simulink library "ComponentLibrary"  (R2017b)
settings: Solver=VariableStepAuto  StartTime=0.0  StopTime=10.0  RelTol=1e-3
undefined symbols (not defined in the file): pelvisPosition, pelvisVelocity, X, Y, Z
libraries: xpcethercatlib x79, sm_lib x21, nesl_utility x13, slrtlib x3, ComponentLibrary x2
(part 2 of 2)

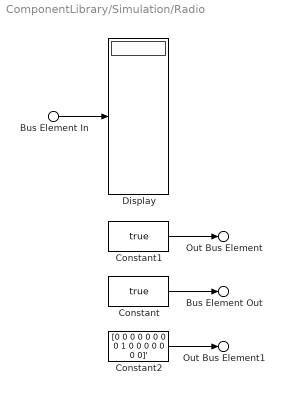
== system ComponentLibrary/Simulation/Radio ==
  Bus Element In : Inport  PortName=InBus  Element=channel
  Constant : Constant  Value=true  OutDataTypeStr=boolean
  Constant1 : Constant  Value=true  OutDataTypeStr=boolean
  Constant2 : Constant  Value=[0 0 0 0 0 0 0 0 1 0 0 0 0 0 0 0]'
  Display : Display
  Out Bus Element : Outport  PortName=OutBus  Element=radioReceiverSignalGood
  Bus Element Out : Outport  PortName=OutBus  Element=receiverMedullaSignalGood
  Out Bus Element1 : Outport  PortName=OutBus  Element=channel
  wires:
  Constant1/1 -> Out Bus Element/1
  Constant2/1 -> Out Bus Element1/1
  Constant/1 -> Bus Element Out/1
  Bus Element In/1 -> Display/1

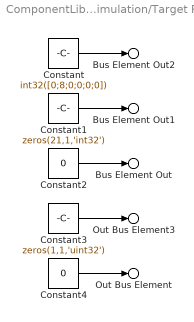
== system ComponentLibrary/Simulation/Target PC ==
  Constant : Constant  Value=int32([0;8;0;0;0;0])
  Constant1 : Constant  Value=zeros(21,1,'int32')
  Constant2 : Constant  Value=0
  Constant3 : Constant  Value=zeros(1,1,'uint32')
  Constant4 : Constant  Value=0
  Bus Element Out2 : Outport  PortName=OutBus  Element=etherCatStatus
  Bus Element Out1 : Outport  PortName=OutBus  Element=etherCatNotifications
  Bus Element Out : Outport  PortName=OutBus  Element=taskExecutionTime
  Out Bus Element3 : Outport  PortName=OutBus  Element=overloadCounter
  Out Bus Element : Outport  PortName=OutBus  Element=cpuTemperature
  wires:
  Constant/1 -> Bus Element Out2/1
  Constant1/1 -> Bus Element Out1/1
  Constant2/1 -> Bus Element Out/1
  Constant4/1 -> Out Bus Element/1
  Constant3/1 -> Out Bus Element3/1

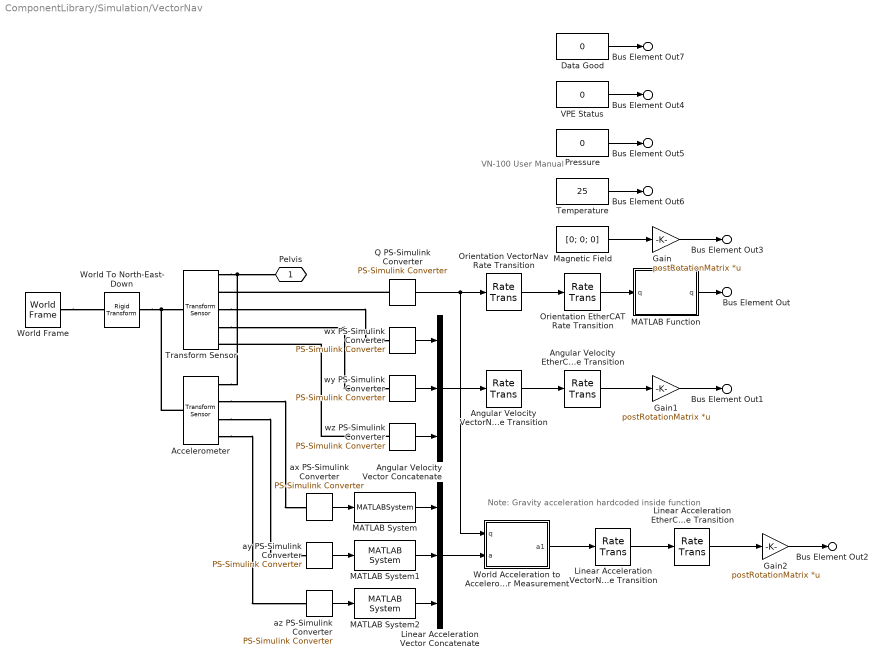
== system ComponentLibrary/Simulation/VectorNav ==
  note: Note: Gravity acceleration hardcoded inside function
  note: VN-100 User Manual
  Accelerometer : sm_lib/Frames and Transforms/Transform Sensor  MeasurementFrame=Base  SenseAngle=off  SenseAxis=off  SenseAngle1=off  SenseAngle2=off  SenseAngle3=off  SenseQ=off  SenseR=off  SenseOmegaX=off  SenseOmegaY=off  SenseOmegaZ=off  SenseOmega1=off  SenseOmega2=off  SenseOmega3=off  SenseQDot=off  SenseRDot=off  SenseAlphaX=off  SenseAlphaY=off  SenseAlphaZ=off  SenseAlpha1=off  SenseAlpha2=off  SenseAlpha3=off  SenseQDDot=off  SenseRDDot=off  SenseX=off  SenseY=off  SenseZ=off  SenseRad=off  SenseAzim=off  SenseDist=off  SenseInc=off  SenseXDot=off  SenseYDot=off  SenseZDot=off  SenseRadDot=off  SenseAzimDot=off  SenseDistDot=off  SenseIncDot=off  SenseXDDot=on  SenseYDDot=on  SenseZDDot=on  SenseRadDDot=off  SenseAzimDDot=off  SenseDistDDot=off  SenseIncDDot=off
  Angular Velocity EtherCAT Rate Transition : RateTransition  Deterministic=off  OutPortSampleTimeOpt=Inherit
  Angular Velocity Vector Concatenate : Concatenate  NumInputs=3
  Angular Velocity VectorNav Rate Transition : RateTransition  Deterministic=off  OutPortSampleTime=VectorNavModule.sampleTime
  Data Good : Constant  Value=0  OutDataTypeStr=boolean
  Gain : Gain  Gain=postRotationMatrix  Multiplication=Matrix(K*u)
  Gain1 : Gain  Gain=postRotationMatrix  Multiplication=Matrix(K*u)
  Gain2 : Gain  Gain=postRotationMatrix  Multiplication=Matrix(K*u)
  Linear Acceleration EtherCAT Rate Transition : RateTransition  Deterministic=off  InitialCondition=[0; 0; 0]  OutPortSampleTimeOpt=Inherit
  Linear Acceleration Vector Concatenate : Concatenate  NumInputs=3
  Linear Acceleration VectorNav Rate Transition : RateTransition  Deterministic=off  InitialCondition=[0; 0; 0]  OutPortSampleTime=VectorNavModule.sampleTime
  MATLAB Function : MATLAB Function  TreatAsAtomicUnit=on
  MATLAB System : MATLABSystem  System=FilterSystem  a=[1 -0.8]  b=0.2  SimulateUsing=Code generation
      mask Type: FilterSystem
      mask Display: disp('Filter');
  MATLAB System1 : ComponentLibrary/Simulation/VectorNav/MATLAB System  a=[1 -0.8]  b=0.2  SimulateUsing=Code generation
  MATLAB System2 : ComponentLibrary/Simulation/VectorNav/MATLAB System  a=[1 -0.8]  b=0.2  SimulateUsing=Code generation
  Magnetic Field : Constant  Value=[0; 0; 0]
  Orientation EtherCAT Rate Transition : RateTransition  Deterministic=off  InitialCondition=[0; 0; 0; 1]  OutPortSampleTimeOpt=Inherit
  Orientation VectorNav Rate Transition : RateTransition  Deterministic=off  InitialCondition=[0; 0; 0; 1]  OutPortSampleTime=VectorNavModule.sampleTime
  Pressure : Constant  Value=0
  Q PS-Simulink Converter : nesl_utility/PS-Simulink Converter  PhysicalDomain=network_engine_domain  SubClassName=ps_output  LeftPortType=input  RightPortType=output  PseudoPeriodic=off  Frequencies=[]  Unit=1  AffineConversion=off
  Temperature : Constant  Value=25
  Transform Sensor : sm_lib/Frames and Transforms/Transform Sensor  MeasurementFrame=Follower  SenseAngle=off  SenseAxis=off  SenseAngle1=off  SenseAngle2=off  SenseAngle3=off  SenseQ=on  SenseR=off  SenseOmegaX=on  SenseOmegaY=on  SenseOmegaZ=on  SenseOmega1=off  SenseOmega2=off  SenseOmega3=off  SenseQDot=off  SenseRDot=off  SenseAlphaX=off  SenseAlphaY=off  SenseAlphaZ=off  SenseAlpha1=off  SenseAlpha2=off  SenseAlpha3=off  SenseQDDot=off  SenseRDDot=off  SenseX=off  SenseY=off  SenseZ=off  SenseRad=off  SenseAzim=off  SenseDist=off  SenseInc=off  SenseXDot=off  SenseYDot=off  SenseZDot=off  SenseRadDot=off  SenseAzimDot=off  SenseDistDot=off  SenseIncDot=off  SenseXDDot=off  SenseYDDot=off  SenseZDDot=off  SenseRadDDot=off  SenseAzimDDot=off  SenseDistDDot=off  SenseIncDDot=off
  VPE Status : Constant  Value=0  OutDataTypeStr=uint16
  World Acceleration to Accelerometer Measurement : MATLAB Function  TreatAsAtomicUnit=on
  World Frame : sm_lib/Frames and Transforms/World Frame
  World To North-East-Down : sm_lib/Frames and Transforms/Rigid Transform  TranslationMethod=None  TranslationStandardOffset=0  TranslationLengthUnit=m  TranslationStandardAxis=+Z  TranslationCartesianOffset=[0 0 0]  TranslationROffset=0  TranslationROffsetUnits=m  TranslationZOffset=0  TranslationZOffsetUnits=m  TranslationThetaOffset=0  TranslationThetaOffsetUnits=deg  RotationMethod=StandardAxis  RotationAngleUnits=deg  RotationStandardAxis=+X  RotationAngle=180  RotationArbitraryAxis=[0 0 1]  FollAlignAxisA=+X  BaseAlignAxisA=+Y  FollAlignAxisB=+Y  BaseAlignAxisB=+Z  RotationSequenceAxes=FollowerAxes  RotationSequence=XYX  RotationSequenceAngles=[0 0 0]  RotationSequenceAnglesUnits=deg  RotationMatrix=[1 0 0; 0 1 0; 0 0 1]
  ax PS-Simulink Converter : nesl_utility/PS-Simulink Converter  PhysicalDomain=network_engine_domain  SubClassName=ps_output  LeftPortType=input  RightPortType=output  PseudoPeriodic=off  Frequencies=[]  Unit=m/s/s  AffineConversion=off
  ay PS-Simulink Converter : nesl_utility/PS-Simulink Converter  PhysicalDomain=network_engine_domain  SubClassName=ps_output  LeftPortType=input  RightPortType=output  PseudoPeriodic=off  Frequencies=[]  Unit=m/s/s  AffineConversion=off
  az PS-Simulink Converter : nesl_utility/PS-Simulink Converter  PhysicalDomain=network_engine_domain  SubClassName=ps_output  LeftPortType=input  RightPortType=output  PseudoPeriodic=off  Frequencies=[]  Unit=m/s/s  AffineConversion=off
  wx PS-Simulink Converter : nesl_utility/PS-Simulink Converter  PhysicalDomain=network_engine_domain  SubClassName=ps_output  LeftPortType=input  RightPortType=output  PseudoPeriodic=off  Frequencies=[]  Unit=1  AffineConversion=off
  wy PS-Simulink Converter : nesl_utility/PS-Simulink Converter  PhysicalDomain=network_engine_domain  SubClassName=ps_output  LeftPortType=input  RightPortType=output  PseudoPeriodic=off  Frequencies=[]  Unit=1  AffineConversion=off
  wz PS-Simulink Converter : nesl_utility/PS-Simulink Converter  PhysicalDomain=network_engine_domain  SubClassName=ps_output  LeftPortType=input  RightPortType=output  PseudoPeriodic=off  Frequencies=[]  Unit=1  AffineConversion=off
  Pelvis : PMIOPort  Port=1  Side=Left
  Bus Element Out7 : Outport  PortName=OutBus  Element=dataGood
  Bus Element Out4 : Outport  PortName=OutBus  Element=vpeStatus
  Bus Element Out5 : Outport  PortName=OutBus  Element=pressure
  Bus Element Out6 : Outport  PortName=OutBus  Element=temperature
  Bus Element Out3 : Outport  PortName=OutBus  Element=magneticField
  Bus Element Out1 : Outport  PortName=OutBus  Element=angularVelocity
  Bus Element Out2 : Outport  PortName=OutBus  Element=linearAcceleration
  Bus Element Out : Outport  PortName=OutBus  Element=orientation
  wires:
  Angular Velocity VectorNav Rate Transition/1 -> Angular Velocity EtherCAT Rate Transition/1
  wz PS-Simulink Converter/1 -> Angular Velocity Vector Concatenate/3
  az PS-Simulink Converter/1 -> MATLAB System2/1
  wx PS-Simulink Converter/1 -> Angular Velocity Vector Concatenate/1
  ax PS-Simulink Converter/1 -> MATLAB System/1
  VPE Status/1 -> Bus Element Out4/1
  Orientation EtherCAT Rate Transition/1 -> MATLAB Function/1("q ")
  Q PS-Simulink Converter/1 -> World Acceleration to Accelerometer Measurement/1(q), Orientation VectorNav Rate Transition/1
  Temperature/1 -> Bus Element Out6/1
  wy PS-Simulink Converter/1 -> Angular Velocity Vector Concatenate/2
  Angular Velocity EtherCAT Rate Transition/1 -> Gain1/1
  Orientation VectorNav Rate Transition/1 -> Orientation EtherCAT Rate Transition/1
  Linear Acceleration EtherCAT Rate Transition/1 -> Gain2/1
  Linear Acceleration VectorNav Rate Transition/1 -> Linear Acceleration EtherCAT Rate Transition/1
  Data Good/1 -> Bus Element Out7/1
  ay PS-Simulink Converter/1 -> MATLAB System1/1
  Magnetic Field/1 -> Gain/1
  Angular Velocity Vector Concatenate/1 -> Angular Velocity VectorNav Rate Transition/1
  Pressure/1 -> Bus Element Out5/1
  Gain/1 -> Bus Element Out3/1
  Gain1/1 -> Bus Element Out1/1
  MATLAB Function/1(q) -> Bus Element Out/1
  MATLAB System/1 -> Linear Acceleration Vector Concatenate/1
  MATLAB System1/1 -> Linear Acceleration Vector Concatenate/2
  MATLAB System2/1 -> Linear Acceleration Vector Concatenate/3
  Gain2/1 -> Bus Element Out2/1
  World Acceleration to Accelerometer Measurement/1(a1) -> Linear Acceleration VectorNav Rate Transition/1
  Linear Acceleration Vector Concatenate/1 -> World Acceleration to Accelerometer Measurement/2(a)
  connections:
  Transform Sensor/RConn4 -- wy PS-Simulink Converter/LConn1
  World To North-East-Down/RConn1 -- Accelerometer/LConn1 -- Transform Sensor/LConn1
  Accelerometer/RConn3 -- ay PS-Simulink Converter/LConn1
  World Frame/RConn1 -- World To North-East-Down/LConn1
  Q PS-Simulink Converter/LConn1 -- Transform Sensor/RConn2
  Accelerometer/RConn2 -- ax PS-Simulink Converter/LConn1
  Transform Sensor/RConn1 -- Pelvis/RConn1 -- Accelerometer/RConn1
  Accelerometer/RConn4 -- az PS-Simulink Converter/LConn1
  Transform Sensor/RConn3 -- wx PS-Simulink Converter/LConn1
  wz PS-Simulink Converter/LConn1 -- Transform Sensor/RConn5

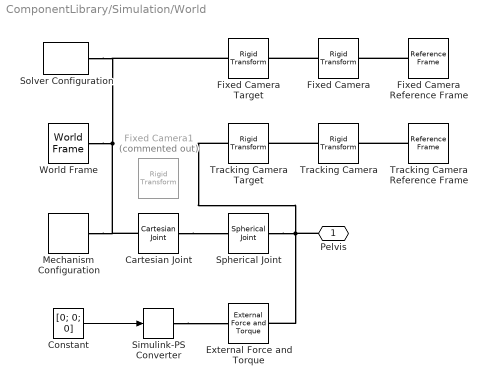
== system ComponentLibrary/Simulation/World ==
  Cartesian Joint : sm_lib/Joints/Cartesian Joint  SenseConstraintForce=off  SenseConstraintForceX=off  SenseConstraintForceY=off  SenseConstraintForceZ=off  SenseConstraintTorque=off  SenseConstraintTorqueX=off  SenseConstraintTorqueY=off  SenseConstraintTorqueZ=off  SenseTotalForce=off  SenseTotalForceX=off  SenseTotalForceY=off  SenseTotalForceZ=off  SenseTotalTorque=off  SenseTotalTorqueX=off  SenseTotalTorqueY=off  SenseTotalTorqueZ=off  CompositeWrenchDir=FollowerOnBase  CompositeWrenchFrame=BaseFrame  PxEquilibriumPosition=0  PxEquilibriumPositionUnits=m  PxSpringStiffness=0  PxSpringStiffnessUnits=N/m  PxDampingCoefficient=0  PxDampingCoefficientUnits=N/(m/s)  PxTorqueActuationMode=NoTorque  PxMotionActuationMode=ComputedMotion  PxSensePosition=off  PxSenseVelocity=off  PxSenseAcceleration=off  PxSenseTorqueForce=off  PxPositionTargetSpecify=on  PxPositionTargetPriority=High  PxPositionTargetValue=pelvisPosition(1)  PxPositionTargetValueUnits=m  PxVelocityTargetSpecify=on  PxVelocityTargetPriority=High  PxVelocityTargetValue=pelvisVelocity(1)  PxVelocityTargetValueUnits=m/s  PyEquilibriumPosition=0  PyEquilibriumPositionUnits=m  PySpringStiffness=0  PySpringStiffnessUnits=N/m  PyDampingCoefficient=0  PyDampingCoefficientUnits=N/(m/s)  PyTorqueActuationMode=NoTorque  PyMotionActuationMode=ComputedMotion  PySensePosition=off  PySenseVelocity=off  PySenseAcceleration=off  PySenseTorqueForce=off  PyPositionTargetSpecify=on  PyPositionTargetPriority=High  PyPositionTargetValue=pelvisPosition(2)  PyPositionTargetValueUnits=m  PyVelocityTargetSpecify=on  PyVelocityTargetPriority=High  PyVelocityTargetValue=pelvisVelocity(2)  PyVelocityTargetValueUnits=m/s  PzEquilibriumPosition=pelvisPosition(3)  PzEquilibriumPositionUnits=m  PzSpringStiffness=5000  PzSpringStiffnessUnits=N/m  PzDampingCoefficient=500  PzDampingCoefficientUnits=N/(m/s)  PzTorqueActuationMode=NoTorque  PzMotionActuationMode=ComputedMotion  PzSensePosition=off  PzSenseVelocity=off  PzSenseAcceleration=off  PzSenseTorqueForce=off  PzPositionTargetSpecify=on  PzPositionTargetPriority=High  PzPositionTargetValue=pelvisPosition(3)  PzPositionTargetValueUnits=m  PzVelocityTargetSpecify=on  PzVelocityTargetPriority=High  PzVelocityTargetValue=pelvisVelocity(3)  PzVelocityTargetValueUnits=m/s
  Constant : Constant  Value=[0; 0; 0]
  External Force and Torque : sm_lib/Forces and Torques/External Force and Torque  ForceResolutionFrame=World  EnableForceX=off  EnableForceY=off  EnableForceZ=off  EnableForce=on  TorqueResolutionFrame=AttachedFrame  EnableTorqueX=off  EnableTorqueY=off  EnableTorqueZ=off  EnableTorque=off
  Fixed Camera : sm_lib/Frames and Transforms/Rigid Transform  TranslationMethod=Cartesian  TranslationStandardOffset=0  TranslationLengthUnit=m  TranslationStandardAxis=+Z  TranslationCartesianOffset=[1.5 -1.5 0.5]  TranslationROffset=0  TranslationROffsetUnits=m  TranslationZOffset=0  TranslationZOffsetUnits=m  TranslationThetaOffset=0  TranslationThetaOffsetUnits=deg  RotationMethod=None  RotationAngleUnits=deg  RotationStandardAxis=+Z  RotationAngle=0.0  RotationArbitraryAxis=[0 0 1]  FollAlignAxisA=+X  BaseAlignAxisA=+Y  FollAlignAxisB=+Y  BaseAlignAxisB=+Z  RotationSequenceAxes=FollowerAxes  RotationSequence=XYX  RotationSequenceAngles=[0 0 0]  RotationSequenceAnglesUnits=deg  RotationMatrix=[1 0 0; 0 1 0; 0 0 1]
  Fixed Camera1 : sm_lib/Frames and Transforms/Rigid Transform  Commented=on  TranslationMethod=Cartesian  TranslationStandardOffset=0  TranslationLengthUnit=m  TranslationStandardAxis=+Z  TranslationCartesianOffset=[pelvisPosition(1),pelvisPosition(2),pelvisPosition(3)]  TranslationROffset=0  TranslationROffsetUnits=m  TranslationZOffset=0  TranslationZOffsetUnits=m  TranslationThetaOffset=0  TranslationThetaOffsetUnits=deg  RotationMethod=None  RotationAngleUnits=deg  RotationStandardAxis=+Z  RotationAngle=0.0  RotationArbitraryAxis=[0 0 1]  FollAlignAxisA=+X  BaseAlignAxisA=+Y  FollAlignAxisB=+Y  BaseAlignAxisB=+Z  RotationSequenceAxes=FollowerAxes  RotationSequence=XYX  RotationSequenceAngles=[0 0 0]  RotationSequenceAnglesUnits=deg  RotationMatrix=[1 0 0; 0 1 0; 0 0 1]
  Fixed Camera Target : sm_lib/Frames and Transforms/Rigid Transform  TranslationMethod=Cartesian  TranslationStandardOffset=0  TranslationLengthUnit=m  TranslationStandardAxis=+Z  TranslationCartesianOffset=[0 0 0.5]  TranslationROffset=0  TranslationROffsetUnits=m  TranslationZOffset=0  TranslationZOffsetUnits=m  TranslationThetaOffset=0  TranslationThetaOffsetUnits=deg  RotationMethod=None  RotationAngleUnits=deg  RotationStandardAxis=+Z  RotationAngle=0.0  RotationArbitraryAxis=[0 0 1]  FollAlignAxisA=+X  BaseAlignAxisA=+Y  FollAlignAxisB=+Y  BaseAlignAxisB=+Z  RotationSequenceAxes=FollowerAxes  RotationSequence=XYX  RotationSequenceAngles=[0 0 0]  RotationSequenceAnglesUnits=deg  RotationMatrix=[1 0 0; 0 1 0; 0 0 1]
  Fixed Camera Reference Frame : sm_lib/Frames and Transforms/Reference Frame
  Mechanism Configuration : sm_lib/Utilities/Mechanism Configuration  UniformGravity=Constant  GravityVector=[0 0 -9.80665]  GravityUnits=m/s^2  LinearizationDelta=0.001
  Simulink-PS Converter : nesl_utility/Simulink-PS Converter  PhysicalDomain=network_engine_domain  SubClassName=ps_input  LeftPortType=input  RightPortType=output  PseudoPeriodic=off  Frequencies=[]  NoiseDistribution=none  NoiseParameters=[]  Unit=1  AffineConversion=off  FilteringAndDerivatives=provide  SimscapeFilterOrder=1  InputFilterTimeConstant=0.001  UdotUserProvided=0
  Solver Configuration : nesl_utility/Solver Configuration  PhysicalDomain=network_engine_domain  SubClassName=solver  LeftPortType=input  RightPortType=generic  Accelerate=off  Tones=[]  Harmonics=[]  SimulateNoise=off  Profile=off  UseLocalSampling=off  EnableSwitchedLinearOptims=on  FrequencyDomain=off  UseCCode=off  RelTol=0.001  AbsTol=1e-06  MinStep=1e-09  ToWorkspace=off  RevertToSquareIcSolve=off  NumHomotopyIterations=100  PhasorMode=off  PhasorModeNumHarmonics=1  DoDC=off  ResidualTolerance=1e-09  UseLocalSolver=off  LocalSolverChoice=NE_BACKWARD_EULER_ADVANCER  LocalSolverSampleTime=0.001  DoFixedCost=off  MaxNonlinIter=3  MaxModeIter=2  LinearAlgebra=Sparse  DelaysMemoryBudget=1024  AutomaticFiltering=on  FilteringTimeConstant=0.001
  Spherical Joint : sm_lib/Joints/Spherical Joint  SenseConstraintForce=off  SenseConstraintForceX=off  SenseConstraintForceY=off  SenseConstraintForceZ=off  SenseConstraintTorque=off  SenseConstraintTorqueX=off  SenseConstraintTorqueY=off  SenseConstraintTorqueZ=off  SenseTotalForce=off  SenseTotalForceX=off  SenseTotalForceY=off  SenseTotalForceZ=off  SenseTotalTorque=off  SenseTotalTorqueX=off  SenseTotalTorqueY=off  SenseTotalTorqueZ=off  CompositeWrenchDir=FollowerOnBase  CompositeWrenchFrame=BaseFrame  DefPosRotationMethod=None  DefPosRotationAngleUnits=deg  DefPosRotationStandardAxis=+Z  DefPosRotationAngle=0.0  DefPosRotationArbitraryAxis=[0 0 1]  DefPosFollAlignAxisA=+X  DefPosBaseAlignAxisA=+Y  DefPosFollAlignAxisB=+Y  DefPosBaseAlignAxisB=+Z  DefPosRotationSequenceAxes=FollowerAxes  DefPosRotationSequence=XYX  DefPosRotationSequenceAngles=[0 0 0]  DefPosRotationSequenceAnglesUnits=deg  DefPosRotationMatrix=[1 0 0; 0 1 0; 0 0 1]  EqPosRotationMethod=None  EqPosRotationAngleUnits=deg  EqPosRotationStandardAxis=+Z  EqPosRotationAngle=0.0  EqPosRotationArbitraryAxis=[0 0 1]  EqPosFollAlignAxisA=+X  EqPosBaseAlignAxisA=+Y  EqPosFollAlignAxisB=+Y  EqPosBaseAlignAxisB=+Z  EqPosRotationSequenceAxes=FollowerAxes  EqPosRotationSequence=XYX  EqPosRotationSequenceAngles=[0 0 0]  EqPosRotationSequenceAnglesUnits=deg  EqPosRotationMatrix=[1 0 0; 0 1 0; 0 0 1]  SpringStiffness=0  SpringStiffnessUnits=N*m/deg  DampingCoefficient=0  DampingCoefficientUnits=N*m/(deg/s)  ActuateTorqueX=off  ActuateTorqueY=off  ActuateTorqueZ=off  ActuateTorque=off  TorqueActuationMode=NoTorque  MotionActuationMode=ComputedMotion  ActuationFrame=BaseFrame  SensePosition=off  SenseVelocityX=off  SenseVelocityY=off  SenseVelocityZ=off  SenseVelocity=off  SenseAccelerationX=off  SenseAccelerationY=off  SenseAccelerationZ=off  SenseAcceleration=off  SenseTorqueX=off  SenseTorqueY=off  SenseTorqueZ=off  SenseTorqueForce=off  SensingFrame=BaseFrame  PositionTargetRotationMethod=RotationMatrix  PositionTargetRotationAngleUnits=deg  PositionTargetRotationStandardAxis=+Z  PositionTargetRotationAngle=0.0  PositionTargetRotationArbitraryAxis=[0 0 1]  PositionTargetFollAlignAxisA=+X  PositionTargetBaseAlignAxisA=+Y  PositionTargetFollAlignAxisB=+Y  PositionTargetBaseAlignAxisB=+Z  PositionTargetRotationSequenceAxes=FollowerAxes  PositionTargetRotationSequence=XYX  PositionTargetRotationSequenceAngles=[0 0 0]  PositionTargetRotationSequenceAnglesUnits=deg  PositionTargetRotationMatrix=pelvisRotation  PositionTargetSpecify=on  PositionTargetPriority=High  VelocityTargetValue=pelvisAngularVelocity  VelocityTargetValueUnits=rad/s  VelocityTargetSpecify=on  VelocityTargetPriority=High  VelocityTargetInFollowerFrame=on
  Tracking Camera : sm_lib/Frames and Transforms/Rigid Transform  TranslationMethod=Cartesian  TranslationStandardOffset=0  TranslationLengthUnit=m  TranslationStandardAxis=+Z  TranslationCartesianOffset=[1.5 -1.5 0.5]  TranslationROffset=0  TranslationROffsetUnits=m  TranslationZOffset=0  TranslationZOffsetUnits=m  TranslationThetaOffset=0  TranslationThetaOffsetUnits=deg  RotationMethod=None  RotationAngleUnits=deg  RotationStandardAxis=+Z  RotationAngle=0.0  RotationArbitraryAxis=[0 0 1]  FollAlignAxisA=+X  BaseAlignAxisA=+Y  FollAlignAxisB=+Y  BaseAlignAxisB=+Z  RotationSequenceAxes=FollowerAxes  RotationSequence=XYX  RotationSequenceAngles=[0 0 0]  RotationSequenceAnglesUnits=deg  RotationMatrix=[1 0 0; 0 1 0; 0 0 1]
  Tracking Camera Target : sm_lib/Frames and Transforms/Rigid Transform  TranslationMethod=Cartesian  TranslationStandardOffset=0  TranslationLengthUnit=m  TranslationStandardAxis=+Z  TranslationCartesianOffset=[0 0 -0.5]  TranslationROffset=0  TranslationROffsetUnits=m  TranslationZOffset=0  TranslationZOffsetUnits=m  TranslationThetaOffset=0  TranslationThetaOffsetUnits=deg  RotationMethod=None  RotationAngleUnits=deg  RotationStandardAxis=+Z  RotationAngle=0.0  RotationArbitraryAxis=[0 0 1]  FollAlignAxisA=+X  BaseAlignAxisA=+Y  FollAlignAxisB=+Y  BaseAlignAxisB=+Z  RotationSequenceAxes=FollowerAxes  RotationSequence=XYX  RotationSequenceAngles=[0 0 0]  RotationSequenceAnglesUnits=deg  RotationMatrix=[1 0 0; 0 1 0; 0 0 1]
  Tracking Camera Reference Frame : sm_lib/Frames and Transforms/Reference Frame
  World Frame : sm_lib/Frames and Transforms/World Frame
  Pelvis : PMIOPort  Port=1  Side=Right
  wires:
  Constant/1 -> Simulink-PS Converter/1
  connections:
  World Frame/RConn1 -- Mechanism Configuration/RConn1 -- Cartesian Joint/LConn1 -- Solver Configuration/RConn1 -- Fixed Camera Target/LConn1
  Tracking Camera Reference Frame/RConn1 -- Tracking Camera/RConn1
  Tracking Camera/LConn1 -- Tracking Camera Target/RConn1
  Fixed Camera Reference Frame/RConn1 -- Fixed Camera/RConn1
  Fixed Camera/LConn1 -- Fixed Camera Target/RConn1
  Simulink-PS Converter/RConn1 -- External Force and Torque/LConn1
  Pelvis/RConn1 -- Spherical Joint/RConn1 -- Tracking Camera Target/LConn1 -- External Force and Torque/RConn1
  Cartesian Joint/RConn1 -- Spherical Joint/LConn1

== matlab function ComponentLibrary/RealTime/Battery/State of Charge Estimator MATLAB Function ==
  data: voltage input; stateOfCharge output; current input
function stateOfCharge = stateOfChargeEstimator(voltage, current)
  stateOfCharge = BatteryModule.stateOfChargeEstimator(voltage, current);
end % stateOfChargeEstimator

== matlab function ComponentLibrary/Simulation/Elmo Drive/MATLAB Function ==
  data: speed input; torque output; torque input; peakTorque parameter; peakSpeed parameter
function torque = fcn(speed, torque, peakTorque, peakSpeed) %#codegen

  % Cap the velocity at the specified limits to avoid extrapolation
  speed = median([-peakSpeed, speed, peakSpeed]);

  % Linear interpolation of speed-torque curve
  torqueLimit = interp1(...
    [0, 0.5*peakSpeed, peakSpeed], ...
    [peakTorque, peakTorque, 0], ...
    abs(speed));

  % Cap the torque command at the specified imits
  torque = median([-torqueLimit, torque, torqueLimit]);
end % fcn

== matlab function ComponentLibrary/RealTime/Battery/ADC to Amperage MATLAB Function ==
  data: adcValue input; A output
function A = adcToAmperage(adcValue) %#codegen
  A = BatteryModule.adcToAmperage(adcValue);
end % adcToAmperage

== matlab function ComponentLibrary/RealTime/Battery/ADC to Celcius MATLAB Function ==
  data: adcValue input; C output
function C = adcToCelcius(adcValue) %#codegen
  C = BatteryModule.adcToCelcius(adcValue);
end % adcToCelcius

== matlab function ComponentLibrary/RealTime/Elmo Drive/Elmo State Machine MATLAB Function ==
  data: statusWord input; controlWord output
function controlWord = stateMachine(statusWord) %#codegen
  controlWord = ElmoModule.stateMachine(statusWord);
end % stateMachine

== matlab function ComponentLibrary/RealTime/Battery/ADC to Voltage MATLAB Function ==
  data: adcValue input; V output
function V = adcToVoltage(adcValue) %#codegen
  V = BatteryModule.adcToVoltage(adcValue);
end % adcToVoltage

== matlab function ComponentLibrary/Simulation/VectorNav/MATLAB Function ==
  data: q input; q output; preRotationMatrix parameter; postRotationMatrix parameter
function q = fcn(q, preRotationMatrix, postRotationMatrix)
  % Construct constant rotation matrix objects
  R0 = coder.const(Rotation3d(preRotationMatrix));
  R2 = coder.const(Rotation3d(postRotationMatrix));
  
  % Convert rotation matrices into constant quaternion objects
  Q0 = coder.const(R0.getQuaternion);
  Q2 = coder.const(R2.getQuaternion);
  
  % Apply pre and post rotations
  Q1 = Q0*Quaternion(q)*Q2;
  
  % Convert quaternion object to double
  q = Q1.getValue;
end % fcn

== matlab function ComponentLibrary/RealTime/VectorNav/MATLAB Function ==
  data: q input; q output; preRotationMatrix parameter; postRotationMatrix parameter
function q = fcn(q, preRotationMatrix, postRotationMatrix)
  % Construct constant rotation matrix objects
  R0 = coder.const(Rotation3d(preRotationMatrix));
  R2 = coder.const(Rotation3d(postRotationMatrix));
  
  % Convert rotation matrices into constant quaternion objects
  Q0 = coder.const(R0.getQuaternion);
  Q2 = coder.const(R2.getQuaternion);
  
  % Apply pre and post rotations
  Q1 = Q0*Quaternion(q)*Q2;
  
  % Convert quaternion object to double
  q = Q1.getValue;
end % fcn

== matlab function ComponentLibrary/RealTime/Elmo Drive/MATLAB Function ==
  data: torqueIn input; torqueOut output; torqueLimit input
function torqueOut = torqueScaling(torqueIn, torqueLimit)
  %TORQUESCALING Normalize torque as required by Elmo drive
  %
  % Description:
  %   This function scales the commanded torque by the torqueScaling factor and
  %   converts it to an int16. The Elmo takes the int16 signal and then rescales
  %   it so that 1000 is equal to its internal torque limit. Because we pull
  %   that internal torque limit from a SDO, we add an extra check in case it is
  %   zero to prevent dividing by zero.
  
  % Copyright 2018 Agility Robotics
  % Author: Mikhail S. Jones
  
  if torqueLimit == 0
    torqueOut = int16(0);
  else
    torqueOut = int16(torqueIn/torqueLimit);
  end % if
end % torqueScaling

== matlab function ComponentLibrary/Simulation/VectorNav/World Acceleration to Accelerometer Measurement ==
  data: q input; a1 output; a input
function a1 = fcn(q, a)
  % Construct quaternion object
  Q = Quaternion(q);
  
  % Add world gravity acceleration to body acceleration
  a1 = Q.getRotation.getValue'*(a + [0; 0; -9.806]);
end % fcn
